simulink model "A2d_D2A_Stream"  (R2017a)
settings: Solver=FixedStepAuto  StartTime=0.0  StopTime=2  FixedStep=Ts  RelTol=1e-3
values from neighbouring files (symbols this model uses):
  b0 = 1    [A2d_D2A_Stream_setup.m]
  b1 = -2*cos(fnn)    [A2d_D2A_Stream_setup.m]
  b2 = 1    [A2d_D2A_Stream_setup.m]
  Ts = 1/Fs    (= 0.001)    [A2d_D2A_Stream_setup.m]
settings Model: Creator=DR_C  LastModifiedBy=Merc
settings SolverCC: AutoInsertRateTranBlk=on

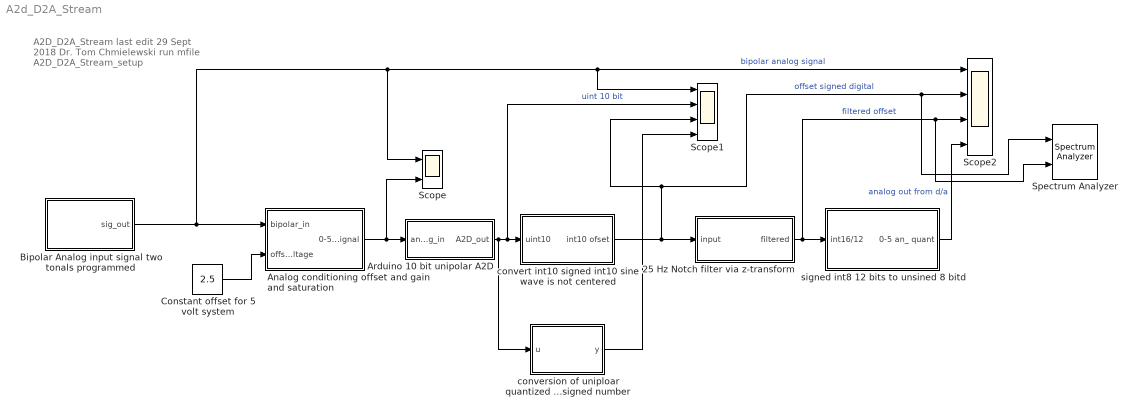
== system A2d_D2A_Stream ==
  note: A2D_D2A_Stream
      | last edit 29 Sept 2018
      | Dr. Tom Chmielewski
      |
      | run mfile A2D_D2A_Stream_setup
  "25 Hz Notch filter via z-transform " : Subsystem
  Analog conditioning offset and gain and saturation : Subsystem
  Arduino 10 bit unipolar A2D : Subsystem
  "Bipolar Analog input signal two tonals programmed " : Subsystem
  Constant offset for 5 volt system : Constant  Value=2.5
  Scope : Scope  NumInputPorts=2
  Scope1 : Scope  NumInputPorts=4
  Scope2 : Scope  NumInputPorts=4
  Spectrum Analyzer : SpectrumAnalyzer  NumInputPorts=2
  conversion of uniploar quantized to floating signed number : MATLAB Function  TreatAsAtomicUnit=on
  convert int10 signed int10 sine wave is not centered : Subsystem
  signed int8 12 bits to unsined 8 bitd : Subsystem
  wires:
  Constant offset for 5 volt system/1 -> Analog conditioning offset and gain and saturation/2(offset_voltage)
  Arduino 10 bit unipolar A2D/1(A2D_out) -> conversion of uniploar quantized to floating signed number/1(u), Scope1/2, convert int10 signed int10 sine wave is not centered/1(uint10)  "uint 10 bit"
  "Bipolar Analog input signal two tonals programmed "/1(sig_out) -> Analog conditioning offset and gain and saturation/1(bipolar_in), Scope/1, Scope2/1, Scope1/1  "bipolar analog signal"
  Analog conditioning offset and gain and saturation/1(0-5V signal) -> Arduino 10 bit unipolar A2D/1(analog_in), Scope/2
  convert int10 signed int10 sine wave is not centered/1(int10 ofset) -> "25 Hz Notch filter via z-transform "/1(input), Scope1/3, Spectrum Analyzer/1, Scope2/2  "offset signed digital"
  conversion of uniploar quantized to floating signed number/1(y) -> Scope1/4
  "25 Hz Notch filter via z-transform "/1("filtered ") -> signed int8 12 bits to unsined 8 bitd/1(int16/12), Spectrum Analyzer/2, Scope2/3  "filtered offset"
  signed int8 12 bits to unsined 8 bitd/1(0-5 an_ quant) -> Scope2/4  "analog out from d/a"

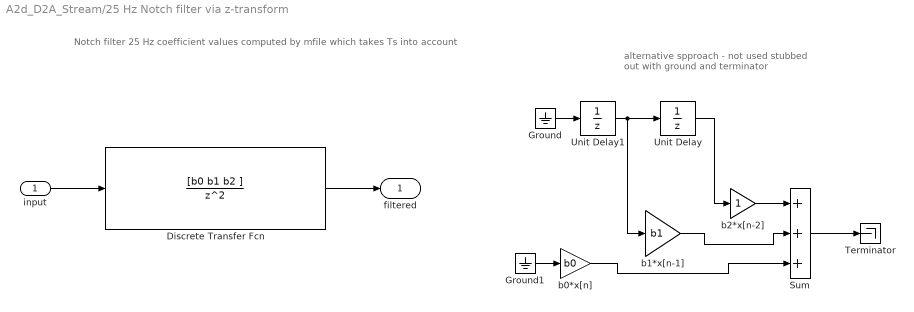
== system A2d_D2A_Stream/25 Hz Notch filter via z-transform  ==
  note: alternative spproach - not used
      | stubbed out with ground and terminator
  note: Notch filter 25 Hz coefficient values computed by mfile which takes Ts into account
  input : Inport
  Discrete Transfer Fcn : DiscreteTransferFcn  Numerator=[b0 b1 b2 ]  Denominator=[1 0 0]
  Ground : Ground
  Ground1 : Ground
  Sum : Sum  Inputs=+++
  Terminator : Terminator
  Unit Delay : UnitDelay  SampleTime=Ts
  Unit Delay1 : UnitDelay  SampleTime=Ts
  b0*x[n] : Gain  Gain=b0
  b1*x[n-1] : Gain  Gain=b1
  b2*x[n-2] : Gain
  "filtered " : Outport
  wires:
  Unit Delay1/1 -> b1*x[n-1]/1, Unit Delay/1
  b0*x[n]/1 -> Sum/3
  b2*x[n-2]/1 -> Sum/1
  b1*x[n-1]/1 -> Sum/2
  Unit Delay/1 -> b2*x[n-2]/1
  input/1 -> Discrete Transfer Fcn/1
  Discrete Transfer Fcn/1 -> "filtered "/1
  Sum/1 -> Terminator/1
  Ground/1 -> Unit Delay1/1
  Ground1/1 -> b0*x[n]/1

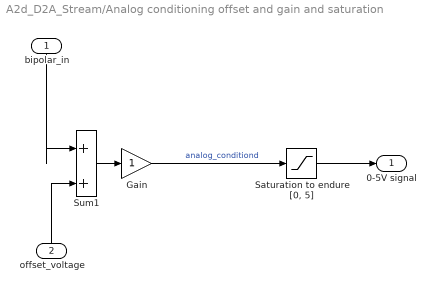
== system A2d_D2A_Stream/Analog conditioning offset and gain and saturation ==
  bipolar_in : Inport
  offset_voltage : Inport  Port=2
  Gain : Gain
  "Saturation to endure [0, 5]" : Saturate  UpperLimit=5.0  LowerLimit=0
  Sum1 : Sum  Inputs=|++
  0-5V signal : Outport
  wires:
  offset_voltage/1 -> Sum1/2
  bipolar_in/1 -> Sum1/1
  Sum1/1 -> Gain/1
  Gain/1 -> "Saturation to endure [0, 5]"/1  "analog_conditiond"
  "Saturation to endure [0, 5]"/1 -> 0-5V signal/1

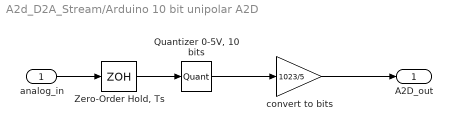
== system A2d_D2A_Stream/Arduino 10 bit unipolar A2D ==
  analog_in : Inport
  "Quantizer 0-5V, 10 bits" : Quantizer  QuantizationInterval=(5/2^10)
  "Zero-Order Hold, Ts" : ZeroOrderHold  SampleTime=Ts
  convert to bits : Gain  Gain=1023/5
  A2D_out : Outport
  wires:
  "Zero-Order Hold, Ts"/1 -> "Quantizer 0-5V, 10 bits"/1
  analog_in/1 -> "Zero-Order Hold, Ts"/1
  "Quantizer 0-5V, 10 bits"/1 -> convert to bits/1
  convert to bits/1 -> A2D_out/1

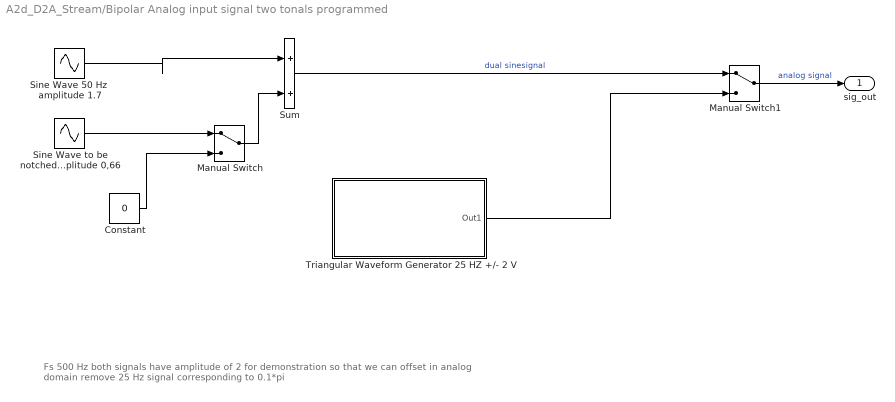
== system A2d_D2A_Stream/Bipolar Analog input signal two tonals programmed  ==
  note: Fs 500 Hz
      | both signals have amplitude of 2 for demonstration so that we can offset in analog domain
      | remove 25 Hz signal corresponding to 0.1*pi
  Constant : Constant  Value=0
  Manual Switch : ManualSwitch
  Manual Switch1 : ManualSwitch
  Sine Wave 50 Hz  amplitude 1.7 : Sin  Amplitude=1.7  Frequency=(2*pi)*50  SampleTime=0
  Sine Wave to be notched Fn 25 Hz analog amplitude 0,66 : Sin  Amplitude=0.66  Frequency=(2*pi)*25  SampleTime=0
  Sum : Sum  Inputs=|++
  Triangular Waveform Generator 25 HZ +/- 2 V : Subsystem
  sig_out : Outport
  wires:
  Sine Wave 50 Hz  amplitude 1.7/1 -> Sum/1
  Sine Wave to be notched Fn 25 Hz analog amplitude 0,66/1 -> Manual Switch/1
  Manual Switch/1 -> Sum/2
  Constant/1 -> Manual Switch/2
  Manual Switch1/1 -> sig_out/1  "analog signal"
  Sum/1 -> Manual Switch1/1  "dual sinesignal"
  Triangular Waveform Generator 25 HZ +/- 2 V/1(Out1) -> Manual Switch1/2

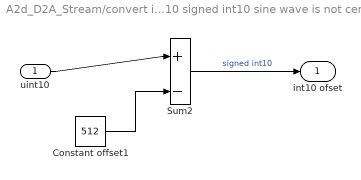
== system A2d_D2A_Stream/convert int10 signed int10 sine wave is not centered ==
  uint10 : Inport
  Constant offset1 : Constant  Value=512
  Sum2 : Sum  Inputs=|+-
  int10 ofset : Outport
  wires:
  uint10/1 -> Sum2/1
  Constant offset1/1 -> Sum2/2
  Sum2/1 -> int10 ofset/1  "signed int10"

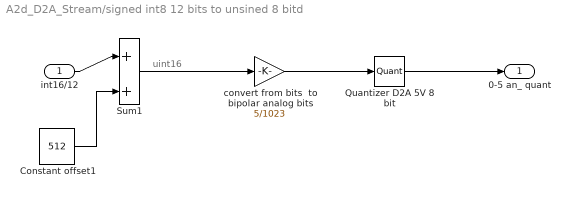
== system A2d_D2A_Stream/signed int8 12 bits to unsined 8 bitd ==
  note: uint16
  int16/12 : Inport
  Constant offset1 : Constant  Value=512
  Quantizer D2A 5V 8 bit : Quantizer  QuantizationInterval=(5/2^8)
  Sum1 : Sum  Inputs=|++
  convert from bits  to bipolar analog bits : Gain  Gain=5/1023
  0-5 an_ quant : Outport
  wires:
  Constant offset1/1 -> Sum1/2
  int16/12/1 -> Sum1/1
  convert from bits  to bipolar analog bits/1 -> Quantizer D2A 5V 8 bit/1
  Quantizer D2A 5V 8 bit/1 -> 0-5 an_ quant/1
  Sum1/1 -> convert from bits  to bipolar analog bits/1

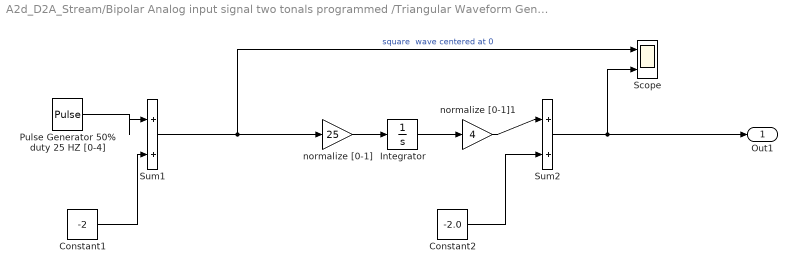
== system A2d_D2A_Stream/Bipolar Analog input signal two tonals programmed /Triangular Waveform Generator 25 HZ +//- 2 V ==
  Constant1 : Constant  Value=-2
  Constant2 : Constant  Value=-2.0
  Integrator : Integrator
  Pulse Generator 50% duty 25 HZ [0-4] : DiscretePulseGenerator  PulseType=Time based  Amplitude=4  Period=1/25  PulseWidth=50
  Scope : Scope  NumInputPorts=2
  Sum1 : Sum  Inputs=|++
  Sum2 : Sum  Inputs=|++
  normalize [0-1] : Gain  Gain=25
  normalize [0-1]1 : Gain  Gain=4
  Out1 : Outport
  wires:
  Sum2/1 -> Scope/2, Out1/1
  Integrator/1 -> normalize [0-1]1/1
  normalize [0-1]/1 -> Integrator/1
  Sum1/1 -> normalize [0-1]/1, Scope/1  "square  wave centered at 0"
  Constant1/1 -> Sum1/2
  Pulse Generator 50% duty 25 HZ [0-4]/1 -> Sum1/1
  Constant2/1 -> Sum2/2
  normalize [0-1]1/1 -> Sum2/1

== matlab function A2d_D2A_Stream/conversion of uniploar quantized to floating signed number ==
  data: u input; y output
function y = fcn(u)
% input is level shifted and quantized analog signal
% this is converted to uint16 to simulate an unsigned 12 bit integer
% then level shifted by 512 and converted to a double 
% at this point the singla procesing is performed
% after signal processing it is converted to an unsigned integeer
% uint8 to perpare for the D/A output

uu = uint16(u); % unsigned 16 bit corrspoinding to q8uantized 0-5 V 
usd = double(uu) - double(512); % signed value
y = usd;
